simulink model "estimator_test_basic"  (R2018b)
settings: Solver=FixedStepAuto  StartTime=0.0  StopTime=1500  FixedStep=sim_params.sample_time_s  MaxStep=sim_params.sample_time_s  MinStep=sim_params.sample_time_s  RelTol=1e-5
undefined symbols (not defined in the file or in its folder): DiscIntNeverNeededParam, fsw_params, gyro_sim_lib, gyroscope_lib, magnetometer_lib, magnetometer_processing_lib, magnetometer_sim_lib, sensor_processing_libs, sim_params, sun_sensor_lib, sunsensor_processing_lib
libraries: vrlib x7, simulink x7, aerolibutil x5, dspmathops x2, simulink_extras x2, extended_kalman_filter_lib x1, ss_vec_2_angles x1, ss_angles_2_vec x1, dynamics_lib x1
settings Model: Creator=Taylor  LastModifiedBy=Taylor
settings SolverCC: InitialStep=sim_params.sample_time_s  InsertRTBMode=Always

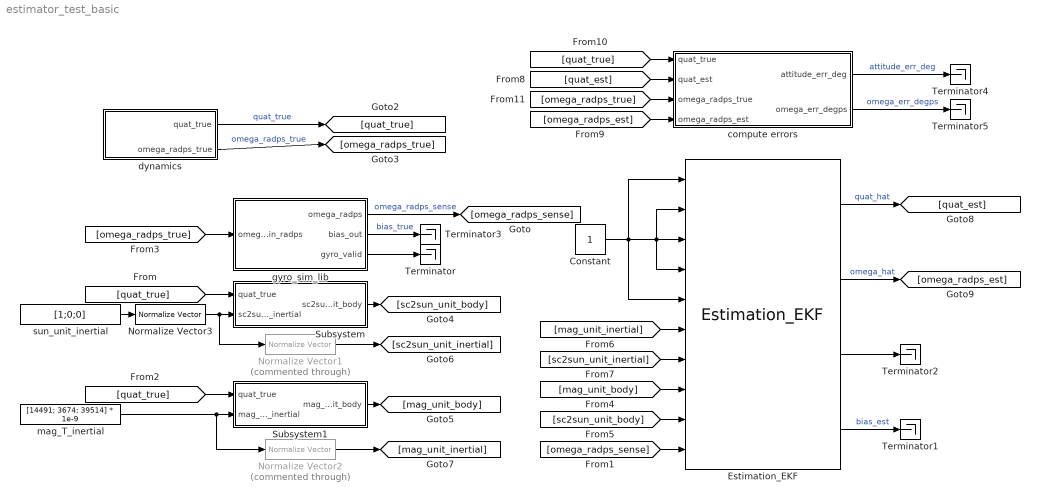
== system estimator_test_basic ==
  Constant : Constant
  "Estimation_EKF " : extended_kalman_filter_lib/Estimation_EKF   SystemSampleTime=-1
  Normalize Vector1 : vrlib/Utilities/Normalize Vector  Commented=through  maxzero=0
      settings: SourceProductName=Simulink 3D Animation  SourceProductBaseCode=VR
  Normalize Vector2 : vrlib/Utilities/Normalize Vector  Commented=through  maxzero=0
      settings: SourceProductName=Simulink 3D Animation  SourceProductBaseCode=VR
  Normalize Vector3 : vrlib/Utilities/Normalize Vector  maxzero=0
      settings: SourceProductName=Simulink 3D Animation  SourceProductBaseCode=VR
  Subsystem : Subsystem
  Subsystem1 : Subsystem
  Terminator{,1..5} (6 alike) : Terminator
  compute errors : Subsystem
  dynamics : Subsystem
  gyro_sim_lib : Subsystem  AncestorBlock=gyroscope_lib/gyro_sim_lib
  "mag_T_inertial " : Constant  Value=[14491; 3674; 39514] * 1e-9
  sun_unit_inertial : Constant  Value=[1;0;0]
  wires:
  Constant/1 -> "Estimation_EKF "/5, "Estimation_EKF "/1, "Estimation_EKF "/2, "Estimation_EKF "/4, "Estimation_EKF "/3
  gyro_sim_lib/1(omega_radps) -> [omega_radps_sense]  "omega_radps_sense"
  [omega_radps_sense] -> "Estimation_EKF "/10
  gyro_sim_lib/2(bias_out) -> Terminator3/1  "bias_true"
  gyro_sim_lib/3(gyro_valid) -> Terminator/1
  Subsystem/1(sc2sun_unit_body) -> [sc2sun_unit_body]
  Subsystem1/1(mag_unit_body) -> [mag_unit_body]
  dynamics/1(quat_true) -> [quat_true]  "quat_true"
  dynamics/2(omega_radps_true) -> [omega_radps_true]  "omega_radps_true"
  [quat_true] -> Subsystem/1(quat_true)
  [quat_true] -> Subsystem1/1(quat_true)
  [omega_radps_true] -> gyro_sim_lib/1(omega_in_radps)
  [mag_unit_body] -> "Estimation_EKF "/8
  [sc2sun_unit_body] -> "Estimation_EKF "/9
  "mag_T_inertial "/1 -> Normalize Vector2/1, Subsystem1/2(mag_T_inertial)
  [mag_unit_inertial] -> "Estimation_EKF "/6
  [sc2sun_unit_inertial] -> "Estimation_EKF "/7
  Normalize Vector1/1 -> [sc2sun_unit_inertial]
  "Estimation_EKF "/2 -> [omega_radps_est]  "omega_hat"
  "Estimation_EKF "/3 -> Terminator2/1
  "Estimation_EKF "/4 -> Terminator1/1  "bias_est"
  [quat_est] -> compute errors/2(quat_est)
  [omega_radps_est] -> compute errors/4(omega_radps_est)
  [quat_true] -> compute errors/1(quat_true)
  [omega_radps_true] -> compute errors/3(omega_radps_true)
  compute errors/1(attitude_err_deg) -> Terminator4/1  "attitude_err_deg"
  compute errors/2(omega_err_degps) -> Terminator5/1  "omega_err_degps"
  "Estimation_EKF "/1 -> [quat_est]  "quat_hat"
  Normalize Vector2/1 -> [mag_unit_inertial]
  Normalize Vector3/1 -> Normalize Vector1/1, Subsystem/2(sc2sun_unit_inertial)
  sun_unit_inertial/1 -> Normalize Vector3/1

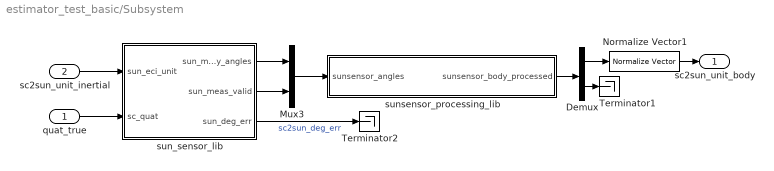
== system estimator_test_basic/Subsystem ==
  quat_true : Inport
  sc2sun_unit_inertial : Inport  Port=2
  Demux : Demux  Outputs=[3 1]
  Mux3 : Mux  Inputs=[2 1]
  Normalize Vector1 : vrlib/Utilities/Normalize Vector  maxzero=0
      settings: SourceProductName=Simulink 3D Animation  SourceProductBaseCode=VR
  Terminator1 : Terminator
  Terminator2 : Terminator
  sun_sensor_lib : Subsystem  AncestorBlock=sun_sensor_lib/sun_sensor_lib
  sunsensor_processing_lib : Subsystem  AncestorBlock=sensor_processing_libs/sunsensor_processing_lib
  sc2sun_unit_body : Outport
  wires:
  quat_true/1 -> sun_sensor_lib/2(sc_quat)
  sc2sun_unit_inertial/1 -> sun_sensor_lib/1(sun_eci_unit)
  sun_sensor_lib/3(sun_deg_err) -> Terminator2/1  "sc2sun_deg_err"
  sunsensor_processing_lib/1(sunsensor_body_processed) -> Demux/1
  sun_sensor_lib/1(sun_meas_body_angles) -> Mux3/1
  Mux3/1 -> sunsensor_processing_lib/1(sunsensor_angles)
  sun_sensor_lib/2(sun_meas_valid) -> Mux3/2
  Demux/1 -> Normalize Vector1/1
  Demux/2 -> Terminator1/1
  Normalize Vector1/1 -> sc2sun_unit_body/1

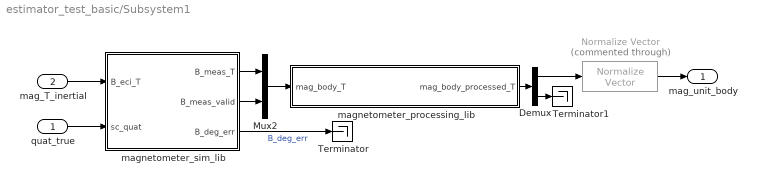
== system estimator_test_basic/Subsystem1 ==
  quat_true : Inport
  mag_T_inertial : Inport  Port=2
  Demux : Demux  Outputs=[3 1]
  Mux2 : Mux  Inputs=[3 1]
  Normalize Vector : vrlib/Utilities/Normalize Vector  Commented=through  maxzero=0
      settings: SourceProductName=Simulink 3D Animation  SourceProductBaseCode=VR
  Terminator : Terminator
  Terminator1 : Terminator
  magnetometer_processing_lib : Subsystem  AncestorBlock=sensor_processing_libs/magnetometer_processing_lib
  magnetometer_sim_lib : Subsystem  AncestorBlock=magnetometer_lib/magnetometer_sim_lib
  mag_unit_body : Outport
  wires:
  quat_true/1 -> magnetometer_sim_lib/2(sc_quat)
  mag_T_inertial/1 -> magnetometer_sim_lib/1(B_eci_T)
  magnetometer_sim_lib/2(B_meas_valid) -> Mux2/2
  magnetometer_sim_lib/1(B_meas_T) -> Mux2/1
  Mux2/1 -> magnetometer_processing_lib/1(mag_body_T)
  magnetometer_sim_lib/3(B_deg_err) -> Terminator/1  "B_deg_err"
  magnetometer_processing_lib/1(mag_body_processed_T) -> Demux/1
  Normalize Vector/1 -> mag_unit_body/1
  Demux/1 -> Normalize Vector/1
  Demux/2 -> Terminator1/1

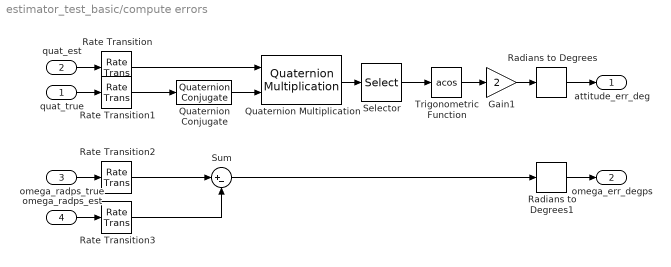
== system estimator_test_basic/compute errors ==
  quat_true : Inport
  quat_est : Inport  Port=2
  omega_radps_true : Inport  Port=3
  omega_radps_est : Inport  Port=4
  Gain1 : Gain  Gain=2
  Quaternion Conjugate : aerolibutil/Quaternion Conjugate
      settings: SourceProductName=Aerospace Blockset  SourceProductBaseCode=AE
  Quaternion Multiplication : aerolibutil/Quaternion Multiplication
  Radians to Degrees : simulink_extras/Transformations/Radians to Degrees
  Radians to Degrees1 : simulink_extras/Transformations/Radians to Degrees
  Rate Transition : RateTransition  InitialCondition=[1;0;0;0]  OutPortSampleTime=fsw_params.estimation.sample_time_s
  Rate Transition1 : RateTransition  InitialCondition=[1;0;0;0]  OutPortSampleTime=fsw_params.estimation.sample_time_s
  Rate Transition2 : RateTransition  OutPortSampleTime=fsw_params.estimation.sample_time_s
  Rate Transition3 : RateTransition  OutPortSampleTime=fsw_params.estimation.sample_time_s
  Selector : Selector  InputPortWidth=4  IndexOptions=Index vector (dialog)  Indices=[1]  OutputSizes=1
  Sum : Sum  Inputs=|+-
  Trigonometric Function : Trigonometry  Operator=acos
  attitude_err_deg : Outport
  omega_err_degps : Outport  Port=2
  wires:
  quat_true/1 -> Rate Transition1/1
  Selector/1 -> Trigonometric Function/1
  Trigonometric Function/1 -> Gain1/1
  Gain1/1 -> Radians to Degrees/1
  Quaternion Multiplication/1 -> Selector/1
  Radians to Degrees/1 -> attitude_err_deg/1
  omega_radps_true/1 -> Rate Transition2/1
  omega_radps_est/1 -> Rate Transition3/1
  Sum/1 -> Radians to Degrees1/1
  Radians to Degrees1/1 -> omega_err_degps/1
  Quaternion Conjugate/1 -> Quaternion Multiplication/2
  quat_est/1 -> Rate Transition/1
  Rate Transition/1 -> Quaternion Multiplication/1
  Rate Transition1/1 -> Quaternion Conjugate/1
  Rate Transition2/1 -> Sum/1
  Rate Transition3/1 -> Sum/2

== system estimator_test_basic/dynamics ==
  Constant : Constant  Commented=on  Value=zeros(3,1)
  Constant1 : Constant  Commented=on  Value=zeros(3,1)
  Constant2 : Constant  Value=[0.1;0;0]
  RigidBodyDynamics : Subsystem  Commented=on  AncestorBlock=dynamics_lib/Dynamics/RigidBodyDynamics
  quat_propagation : dynamics_lib/Dynamics/quat_propagation  SystemSampleTime=-1
  quat_true : Outport
  omega_radps_true : Outport  Port=2
  wires:
  quat_propagation/1 -> quat_true/1
  Constant/1 -> RigidBodyDynamics/1(external_torque)
  Constant1/1 -> RigidBodyDynamics/2(RW_torque)
  Constant2/1 -> omega_radps_true/1, quat_propagation/1

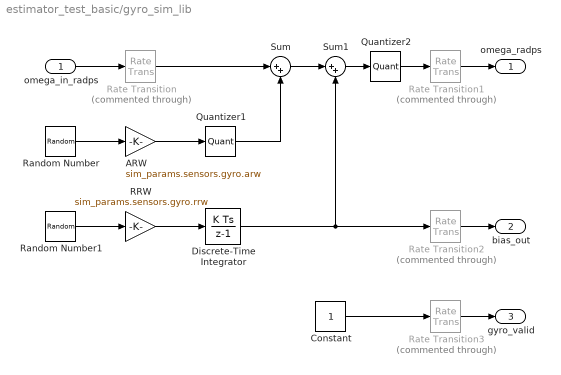
== system estimator_test_basic/gyro_sim_lib ==
  omega_in_radps : Inport
  ARW : Gain  Gain=sim_params.sensors.gyro.arw
  Constant : Constant  SampleTime=sim_params.sensors.gyro.sample_time_s
  Discrete-Time Integrator : DiscreteIntegrator  InitialCondition=sim_params.sensors.gyro.bias_init  SampleTime=-1  ICPrevOutput=DiscIntNeverNeededParam  ICPrevScaledInput=DiscIntNeverNeededParam
  Quantizer1 : Quantizer  QuantizationInterval=sim_params.sensors.gyro.resolution
  Quantizer2 : Quantizer  QuantizationInterval=sim_params.sensors.gyro.resolution
  RRW : Gain  Gain=sim_params.sensors.gyro.rrw
  Random Number : RandomNumber  Mean=[0 0 0]  Variance=[1 1 1]  Seed=[77 88 99]  SampleTime=sim_params.sensors.gyro.sample_time_s
  Random Number1 : RandomNumber  Mean=[0 0 0]  Variance=[1 1 1]  Seed=[81 82 83]  SampleTime=sim_params.sensors.gyro.sample_time_s
  Rate Transition : RateTransition  Commented=through  InitialCondition=sim_params.dynamics.ic.rate_init  OutPortSampleTime=sim_params.sensors.gyro.sample_time_s
  Rate Transition1 : RateTransition  Commented=through  InitialCondition=sim_params.dynamics.ic.rate_init
  Rate Transition2 : RateTransition  Commented=through  InitialCondition=sim_params.sensors.gyro.bias_init
  Rate Transition3 : RateTransition  Commented=through  InitialCondition=1
  Sum : Sum  Inputs=|++
  Sum1 : Sum  Inputs=|++
  omega_radps : Outport
  bias_out : Outport  Port=2
  gyro_valid : Outport  Port=3
  wires:
  Rate Transition3/1 -> gyro_valid/1
  Rate Transition2/1 -> bias_out/1
  Rate Transition1/1 -> omega_radps/1
  Rate Transition/1 -> Sum/1
  Quantizer2/1 -> Rate Transition1/1
  Sum1/1 -> Quantizer2/1
  Discrete-Time Integrator/1 -> Sum1/2, Rate Transition2/1
  Constant/1 -> Rate Transition3/1
  RRW/1 -> Discrete-Time Integrator/1
  Sum/1 -> Sum1/1
  omega_in_radps/1 -> Rate Transition/1
  ARW/1 -> Quantizer1/1
  Random Number1/1 -> RRW/1
  Random Number/1 -> ARW/1
  Quantizer1/1 -> Sum/2

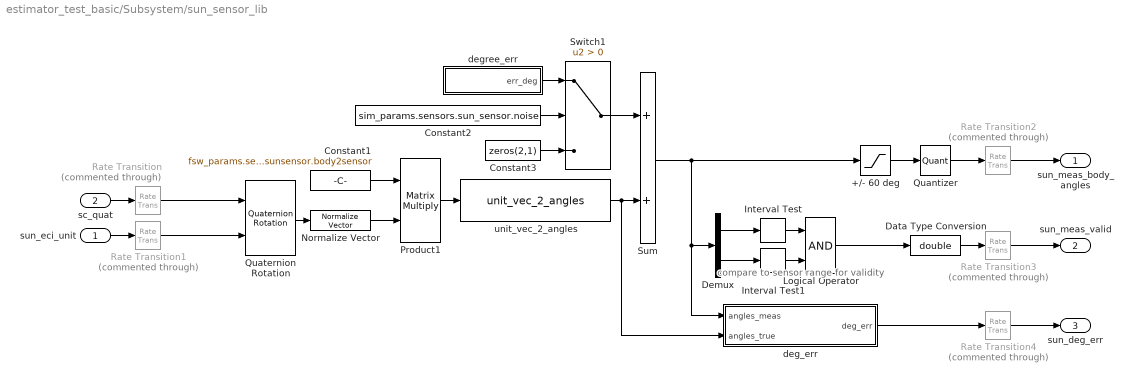
== system estimator_test_basic/Subsystem/sun_sensor_lib ==
  note: compare to sensor range for validity
  sun_eci_unit : Inport
  sc_quat : Inport  Port=2
  +/- 60 deg : Saturate  UpperLimit=60  LowerLimit=-60
  Constant1 : Constant  Value=fsw_params.sensor_processing.sunsensor.body2sensor  SampleTime=sim_params.sensors.sun_sensor.sample_time_s
  Constant2 : Constant  Value=sim_params.sensors.sun_sensor.noise  SampleTime=sim_params.sensors.sun_sensor.sample_time_s
  Constant3 : Constant  Value=zeros(2,1)  SampleTime=sim_params.sensors.sun_sensor.sample_time_s
  Data Type Conversion : DataTypeConversion  OutDataTypeStr=double
  Demux : Demux  Outputs=2
  Interval Test : simulink/Logic and Bit Operations/Interval Test  IntervalClosedRight=on  uplimit=sim_params.sensors.sun_sensor.range_deg  IntervalClosedLeft=on  lowlimit=-sim_params.sensors.sun_sensor.range_deg  OutDataTypeStr=boolean
  Interval Test1 : simulink/Logic and Bit Operations/Interval Test  IntervalClosedRight=on  uplimit=sim_params.sensors.sun_sensor.range_deg  IntervalClosedLeft=on  lowlimit=-sim_params.sensors.sun_sensor.range_deg  OutDataTypeStr=boolean
  Logical Operator : Logic  AllPortsSameDT=off  OutDataTypeStr=boolean
  Normalize Vector : vrlib/Utilities/Normalize Vector  maxzero=0
      settings: SourceProductName=Simulink 3D Animation  SourceProductBaseCode=VR
  Product1 : Product  Multiplication=Matrix(*)  RndMeth=Zero
  Quantizer : Quantizer  QuantizationInterval=sim_params.sensors.sun_sensor.resolution
  Quaternion Rotation : aerolibutil/Quaternion Rotation
  Rate Transition : RateTransition  Commented=through  InitialCondition=sim_params.dynamics.ic.quat_init  OutPortSampleTime=sim_params.sensors.sun_sensor.sample_time_s
  Rate Transition1 : RateTransition  Commented=through  OutPortSampleTime=sim_params.sensors.sun_sensor.sample_time_s
  Rate Transition2 : RateTransition  Commented=through
  Rate Transition3 : RateTransition  Commented=through
  Rate Transition4 : RateTransition  Commented=through
  Sum : Sum
  Switch1 : Switch  Criteria=u2 > Threshold
  deg_err : Subsystem
  degree_err : Subsystem
  unit_vec_2_angles : ss_vec_2_angles/unit_vec_2_angles  SystemSampleTime=-1
  sun_meas_body_angles : Outport
  sun_meas_valid : Outport  Port=2
  sun_deg_err : Outport  Port=3
  wires:
  Rate Transition4/1 -> sun_deg_err/1
  Rate Transition3/1 -> sun_meas_valid/1
  Rate Transition2/1 -> sun_meas_body_angles/1
  Rate Transition1/1 -> Quaternion Rotation/2
  Rate Transition/1 -> Quaternion Rotation/1
  Data Type Conversion/1 -> Rate Transition3/1
  Demux/2 -> Interval Test1/1
  Sum/1 -> Demux/1, deg_err/1(angles_meas), +/- 60 deg/1
  unit_vec_2_angles/1 -> Sum/2, deg_err/2(angles_true)
  Product1/1 -> unit_vec_2_angles/1
  Constant1/1 -> Product1/1
  +/- 60 deg/1 -> Quantizer/1
  Logical Operator/1 -> Data Type Conversion/1
  Interval Test1/1 -> Logical Operator/2
  Interval Test/1 -> Logical Operator/1
  Demux/1 -> Interval Test/1
  Normalize Vector/1 -> Product1/2
  Quantizer/1 -> Rate Transition2/1
  Quaternion Rotation/1 -> Normalize Vector/1
  degree_err/1("err_deg ") -> Switch1/1
  deg_err/1(deg_err) -> Rate Transition4/1
  sun_eci_unit/1 -> Rate Transition1/1
  Switch1/1 -> Sum/1
  Constant3/1 -> Switch1/3
  Constant2/1 -> Switch1/2
  sc_quat/1 -> Rate Transition/1

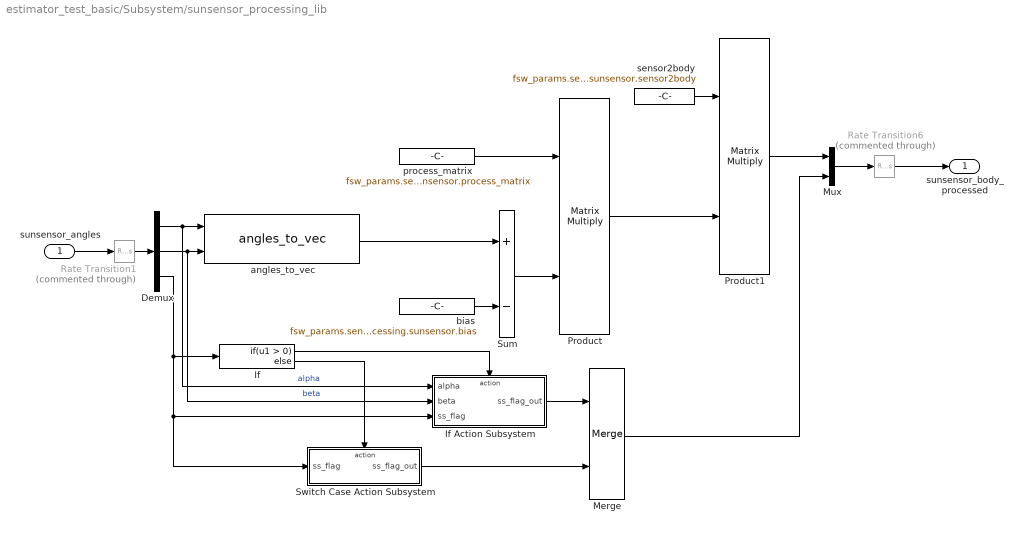
== system estimator_test_basic/Subsystem/sunsensor_processing_lib ==
  sunsensor_angles : Inport
  Demux : Demux  Outputs=[1 1 1]
  If : If
  If Action Subsystem : Subsystem  TreatAsAtomicUnit=on
  Merge : Merge
  Mux : Mux  Inputs=[3 1]
  Product : Product  Multiplication=Matrix(*)
  Product1 : Product  Multiplication=Matrix(*)
  Rate Transition1 : RateTransition  Commented=through  InitialCondition=fsw_params.sensor_processing.sunsensor.ic.angles  OutPortSampleTime=fsw_params.sensor_processing.sunsensor.sample_time_s
  Rate Transition6 : RateTransition  Commented=through
  Sum : Sum  Inputs=+-
  Switch Case Action Subsystem : Subsystem  TreatAsAtomicUnit=on
  angles_to_vec : ss_angles_2_vec/angles_to_vec  SystemSampleTime=-1
  bias : Constant  Value=fsw_params.sensor_processing.sunsensor.bias  SampleTime=fsw_params.sensor_processing.sunsensor.sample_time_s
  process_matrix : Constant  Value=fsw_params.sensor_processing.sunsensor.process_matrix  SampleTime=fsw_params.sensor_processing.sunsensor.sample_time_s
  sensor2body : Constant  Value=fsw_params.sensor_processing.sunsensor.sensor2body  SampleTime=fsw_params.sensor_processing.sunsensor.sample_time_s
  sunsensor_body_processed : Outport
  wires:
  process_matrix/1 -> Product/1
  Sum/1 -> Product/2
  Product/1 -> Product1/2
  bias/1 -> Sum/2
  sunsensor_angles/1 -> Rate Transition1/1
  sensor2body/1 -> Product1/1
  Product1/1 -> Mux/1
  Mux/1 -> Rate Transition6/1
  Rate Transition1/1 -> Demux/1
  Rate Transition6/1 -> sunsensor_body_processed/1
  Demux/1 -> If Action Subsystem/1(alpha), angles_to_vec/1  "alpha"
  Demux/2 -> If Action Subsystem/2(beta), angles_to_vec/2  "beta"
  angles_to_vec/1 -> Sum/1
  Merge/1 -> Mux/2
  Demux/3 -> If Action Subsystem/3(ss_flag), Switch Case Action Subsystem/1(ss_flag), If/1
  If/1 -> If Action Subsystem/Action
  If/2 -> Switch Case Action Subsystem/Action
  If Action Subsystem/1(ss_flag_out) -> Merge/1
  Switch Case Action Subsystem/1(ss_flag_out) -> Merge/2

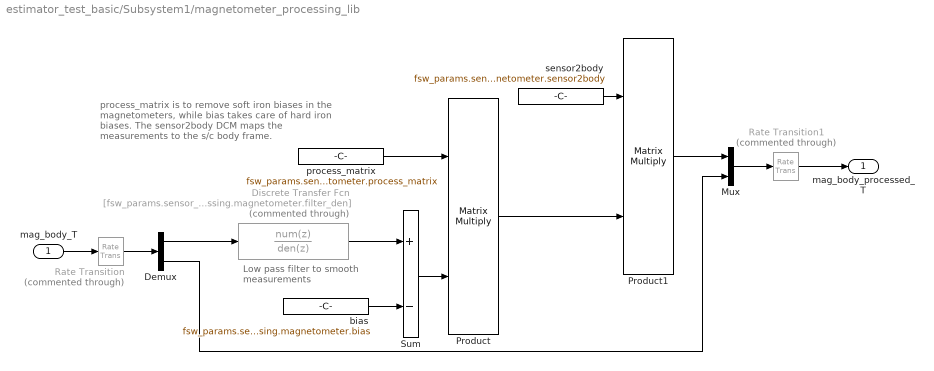
== system estimator_test_basic/Subsystem1/magnetometer_processing_lib ==
  note: Low pass filter to
      | smooth measurements
  note: process_matrix is to remove soft iron
      | biases in the magnetometers, while
      | bias takes care of hard iron biases.
      |
      | The sensor2body DCM maps the
      | measurements to the s/c body
      | frame.
  mag_body_T : Inport
  Demux : Demux  Outputs=[3 1]
  Discrete Transfer Fcn : DiscreteTransferFcn  Commented=through  Numerator=[fsw_params.sensor_processing.magnetometer.filter_num]  Denominator=[1 fsw_params.sensor_processing.magnetometer.filter_den]
  Mux : Mux  Inputs=[3 1]
  Product : Product  Multiplication=Matrix(*)
  Product1 : Product  Multiplication=Matrix(*)
  Rate Transition : RateTransition  Commented=through  OutPortSampleTime=fsw_params.sensor_processing.magnetometer.sample_time_s
  Rate Transition1 : RateTransition  Commented=through
  Sum : Sum  Inputs=+-
  bias : Constant  Value=fsw_params.sensor_processing.magnetometer.bias  SampleTime=fsw_params.sensor_processing.magnetometer.sample_time_s
  process_matrix : Constant  Value=fsw_params.sensor_processing.magnetometer.process_matrix  SampleTime=fsw_params.sensor_processing.magnetometer.sample_time_s
  sensor2body : Constant  Value=fsw_params.sensor_processing.magnetometer.sensor2body  SampleTime=fsw_params.sensor_processing.magnetometer.sample_time_s
  mag_body_processed_T : Outport
  wires:
  Discrete Transfer Fcn/1 -> Sum/1
  Rate Transition1/1 -> mag_body_processed_T/1
  Rate Transition/1 -> Demux/1
  Product1/1 -> Mux/1
  sensor2body/1 -> Product1/1
  Product/1 -> Product1/2
  Mux/1 -> Rate Transition1/1
  Demux/2 -> Mux/2
  Demux/1 -> Discrete Transfer Fcn/1
  process_matrix/1 -> Product/1
  Sum/1 -> Product/2
  bias/1 -> Sum/2
  mag_body_T/1 -> Rate Transition/1

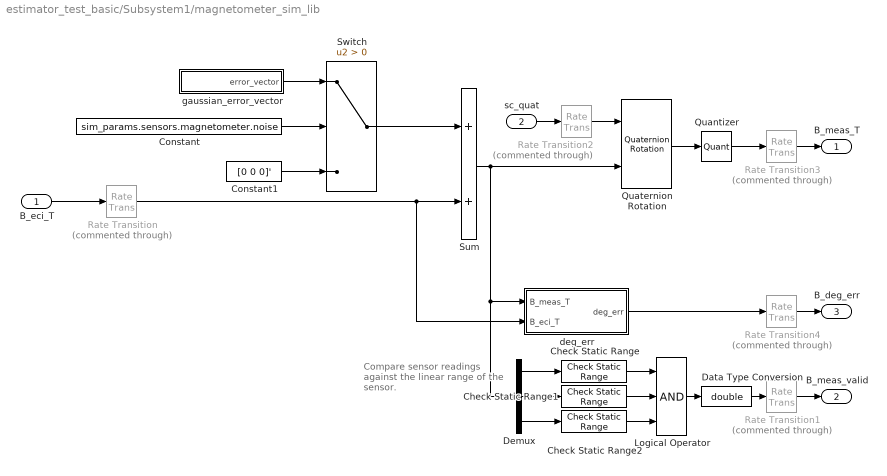
== system estimator_test_basic/Subsystem1/magnetometer_sim_lib ==
  note: Compare sensor readings
      | against the linear range
      | of the sensor.
  B_eci_T : Inport
  sc_quat : Inport  Port=2
  Check Static Range : simulink/Model Verification/Check  Static Range  Description=sim_params.sensors.magnetometer.B_min <= u <= sim_params.sensors.magnetometer.B_max  max=sim_params.sensors.magnetometer.B_max  max_included=on  min=sim_params.sensors.magnetometer.B_min  min_included=on  enabled=on  stopWhenAssertionFail=off  export=on  icon=text
      settings: SourceProductName=Simulink  SourceProductBaseCode=SL
  Check Static Range1 : simulink/Model Verification/Check  Static Range  Description=sim_params.sensors.magnetometer.B_min <= u <= sim_params.sensors.magnetometer.B_max  max=sim_params.sensors.magnetometer.B_max  max_included=on  min=sim_params.sensors.magnetometer.B_min  min_included=on  enabled=on  stopWhenAssertionFail=off  export=on  icon=graphic
      settings: SourceProductName=Simulink  SourceProductBaseCode=SL
  Check Static Range2 : simulink/Model Verification/Check  Static Range  Description=sim_params.sensors.magnetometer.B_min <= u <= sim_params.sensors.magnetometer.B_max  max=sim_params.sensors.magnetometer.B_max  max_included=on  min=sim_params.sensors.magnetometer.B_min  min_included=on  enabled=on  stopWhenAssertionFail=off  export=on  icon=graphic
      settings: SourceProductName=Simulink  SourceProductBaseCode=SL
  Constant : Constant  Value=sim_params.sensors.magnetometer.noise  SampleTime=sim_params.sensors.magnetometer.sample_time_s
  Constant1 : Constant  Value=[0 0 0]'  SampleTime=sim_params.sensors.magnetometer.sample_time_s
  Data Type Conversion : DataTypeConversion  OutDataTypeStr=double
  Demux : Demux  Outputs=3
  Logical Operator : Logic  Inputs=3  AllPortsSameDT=off  OutDataTypeStr=boolean
  Quantizer : Quantizer  QuantizationInterval=sim_params.sensors.magnetometer.resolution
  Quaternion Rotation : aerolibutil/Quaternion Rotation
  Rate Transition : RateTransition  Commented=through  InitialCondition=sim_params.environment.magnetic.ic.eci_T  OutPortSampleTime=sim_params.sensors.magnetometer.sample_time_s
  Rate Transition1 : RateTransition  Commented=through
  Rate Transition2 : RateTransition  Commented=through  InitialCondition=sim_params.dynamics.ic.quat_init  OutPortSampleTime=sim_params.sensors.magnetometer.sample_time_s
  Rate Transition3 : RateTransition  Commented=through  InitialCondition=sim_params.environment.magnetic.ic.eci_T
  Rate Transition4 : RateTransition  Commented=through
  Sum : Sum
  Switch : Switch  Criteria=u2 > Threshold
  deg_err : Subsystem
  gaussian_error_vector : Subsystem
  B_meas_T : Outport
  B_meas_valid : Outport  Port=2
  B_deg_err : Outport  Port=3
  wires:
  Data Type Conversion/1 -> Rate Transition1/1
  Logical Operator/1 -> Data Type Conversion/1
  Check Static Range2/1 -> Logical Operator/3
  Check Static Range1/1 -> Logical Operator/2
  Check Static Range/1 -> Logical Operator/1
  Demux/3 -> Check Static Range2/1
  Demux/2 -> Check Static Range1/1
  Demux/1 -> Check Static Range/1
  Quantizer/1 -> Rate Transition3/1
  Rate Transition4/1 -> B_deg_err/1
  Quaternion Rotation/1 -> Quantizer/1
  Rate Transition3/1 -> B_meas_T/1
  Rate Transition2/1 -> Quaternion Rotation/1
  Rate Transition1/1 -> B_meas_valid/1
  Rate Transition/1 -> Sum/2, deg_err/2(B_eci_T)
  deg_err/1(deg_err) -> Rate Transition4/1
  B_eci_T/1 -> Rate Transition/1
  gaussian_error_vector/1(error_vector) -> Switch/1
  Constant1/1 -> Switch/3
  Sum/1 -> Demux/1, deg_err/1(B_meas_T), Quaternion Rotation/2
  Constant/1 -> Switch/2
  Switch/1 -> Sum/1
  sc_quat/1 -> Rate Transition2/1

== system estimator_test_basic/dynamics/RigidBodyDynamics ==
  external_torque : Inport
  RW_torque : Inport  Port=2
  Discrete-Time Integrator : DiscreteIntegrator  InitialCondition=[0;0;0]  SampleTime=-1  ICPrevOutput=DiscIntNeverNeededParam  ICPrevScaledInput=DiscIntNeverNeededParam
  "Discrete-Time Integrator " : DiscreteIntegrator  InitialCondition=[0.1;0.05;-0.07]  SampleTime=-1  ICPrevOutput=DiscIntNeverNeededParam  ICPrevScaledInput=DiscIntNeverNeededParam
  dynamics : Subsystem
  body_rates : Outport
  wires:
  RW_torque/1 -> dynamics/2(rw_torque_Nm), Discrete-Time Integrator/1
  Discrete-Time Integrator/1 -> dynamics/3(rw_momentum_Nms)
  "Discrete-Time Integrator "/1 -> body_rates/1, dynamics/4(omega_radps)
  external_torque/1 -> dynamics/1(external_torque_Nm)
  dynamics/1(omega_dot) -> "Discrete-Time Integrator "/1

== system estimator_test_basic/Subsystem/sun_sensor_lib/deg_err ==
  note: Computes the norm of the 2x1 degree error vector
  angles_meas : Inport
  angles_true : Inport  Port=2
  Dot Product : DotProduct  InputSameDT=on  OutDataTypeStr=Inherit: Inherit via internal rule
  Sqrt : Sqrt  SaturateOnIntegerOverflow=on
  Sum : Sum  Inputs=+-
  deg_err : Outport
  wires:
  Sqrt/1 -> deg_err/1
  Dot Product/1 -> Sqrt/1
  Sum/1 -> Dot Product/1, Dot Product/2
  angles_true/1 -> Sum/2
  angles_meas/1 -> Sum/1

== system estimator_test_basic/Subsystem/sun_sensor_lib/degree_err ==
  Mux : Mux  Inputs=2
  Random Number2 : RandomNumber  Variance=sim_params.sensors.sun_sensor.deg_err  Seed=51  SampleTime=sim_params.sensors.sun_sensor.sample_time_s
  Random Number3 : RandomNumber  Variance=sim_params.sensors.sun_sensor.deg_err  Seed=52  SampleTime=sim_params.sensors.sun_sensor.sample_time_s
  "err_deg " : Outport
  wires:
  Mux/1 -> "err_deg "/1
  Random Number3/1 -> Mux/2
  Random Number2/1 -> Mux/1

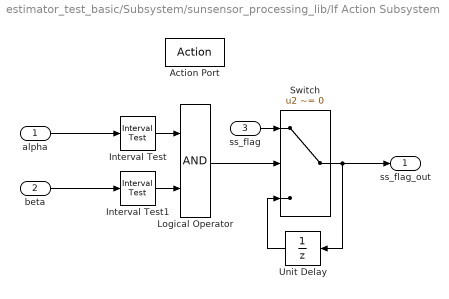
== system estimator_test_basic/Subsystem/sunsensor_processing_lib/If Action Subsystem ==
  alpha : Inport
  beta : Inport  Port=2
  ss_flag : Inport  Port=3
  Action Port : ActionPort  InitializeStates=reset  ActionType=then
  Interval Test : simulink/Logic and Bit Operations/Interval Test  IntervalClosedRight=on  uplimit=fsw_params.sensor_processing.sunsensor.ang_thresh  IntervalClosedLeft=on  lowlimit=-fsw_params.sensor_processing.sunsensor.ang_thresh  OutDataTypeStr=boolean
  Interval Test1 : simulink/Logic and Bit Operations/Interval Test  IntervalClosedRight=on  uplimit=fsw_params.sensor_processing.sunsensor.ang_thresh  IntervalClosedLeft=on  lowlimit=-fsw_params.sensor_processing.sunsensor.ang_thresh  OutDataTypeStr=boolean
  Logical Operator : Logic  AllPortsSameDT=off  OutDataTypeStr=boolean
  Switch : Switch  Criteria=u2 ~= 0
  Unit Delay : UnitDelay  InitialCondition=2  SampleTime=-1
  ss_flag_out : Outport
  wires:
  Switch/1 -> ss_flag_out/1, Unit Delay/1
  Interval Test/1 -> Logical Operator/1
  Interval Test1/1 -> Logical Operator/2
  beta/1 -> Interval Test1/1
  alpha/1 -> Interval Test/1
  ss_flag/1 -> Switch/1
  Logical Operator/1 -> Switch/2
  Unit Delay/1 -> Switch/3

== system estimator_test_basic/Subsystem/sunsensor_processing_lib/Switch Case Action Subsystem ==
  ss_flag : Inport
  Action Port : ActionPort  ActionType=else
  ss_flag_out : Outport
  wires:
  ss_flag/1 -> ss_flag_out/1

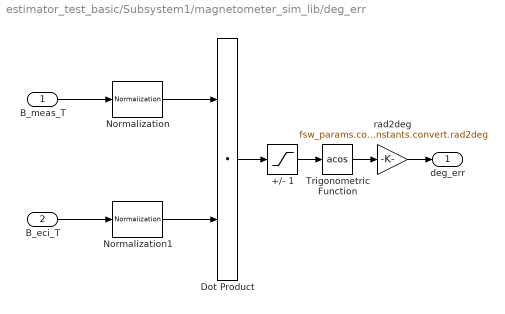
== system estimator_test_basic/Subsystem1/magnetometer_sim_lib/deg_err ==
  B_meas_T : Inport
  B_eci_T : Inport  Port=2
  +/- 1 : Saturate  UpperLimit=1  LowerLimit=-1
  Dot Product : DotProduct  InputSameDT=on  OutDataTypeStr=Inherit: Inherit via internal rule
  Normalization : dspmathops/Normalization  NormType=2-norm  Bias=1e-10  NormOver=Each column  Dimension=1  roundingMode=Floor  overflowMode=off  accumDataTypeStr=Inherit: Same as product output  accumLastDataTypeStr=Inherit: Same as product output  outputDataTypeStr=Inherit: Same as product output  outputMin=[]  outputMax=[]  outputLastDataTypeStr=Inherit: Same as product output
      settings: SourceProductName=DSP System Toolbox
  Normalization1 : dspmathops/Normalization  NormType=2-norm  Bias=1e-10  NormOver=Each column  Dimension=1  roundingMode=Floor  overflowMode=off  accumDataTypeStr=Inherit: Same as product output  accumLastDataTypeStr=Inherit: Same as product output  outputDataTypeStr=Inherit: Same as product output  outputMin=[]  outputMax=[]  outputLastDataTypeStr=Inherit: Same as product output
      settings: SourceProductName=DSP System Toolbox
  Trigonometric Function : Trigonometry  Operator=acos
  rad2deg : Gain  Gain=fsw_params.constants.convert.rad2deg
  deg_err : Outport
  wires:
  rad2deg/1 -> deg_err/1
  +/- 1/1 -> Trigonometric Function/1
  Trigonometric Function/1 -> rad2deg/1
  Dot Product/1 -> +/- 1/1
  Normalization1/1 -> Dot Product/2
  B_eci_T/1 -> Normalization1/1
  Normalization/1 -> Dot Product/1
  B_meas_T/1 -> Normalization/1

== system estimator_test_basic/Subsystem1/magnetometer_sim_lib/gaussian_error_vector ==
  Mux : Mux  Inputs=3
  Random Number2 : RandomNumber  Seed=4  SampleTime=sim_params.sensors.magnetometer.sample_time_s
  Random Number3 : RandomNumber  Seed=5  SampleTime=sim_params.sensors.magnetometer.sample_time_s
  Random Number4 : RandomNumber  Seed=6  SampleTime=sim_params.sensors.magnetometer.sample_time_s
  sigma_mag_x : Gain  Gain=sim_params.sensors.magnetometer.err_x
  sigma_mag_y : Gain  Gain=sim_params.sensors.magnetometer.err_y
  sigma_mag_z : Gain  Gain=sim_params.sensors.magnetometer.err_z
  error_vector : Outport
  wires:
  sigma_mag_z/1 -> Mux/3
  Mux/1 -> error_vector/1
  sigma_mag_y/1 -> Mux/2
  sigma_mag_x/1 -> Mux/1
  Random Number3/1 -> sigma_mag_y/1
  Random Number4/1 -> sigma_mag_z/1
  Random Number2/1 -> sigma_mag_x/1

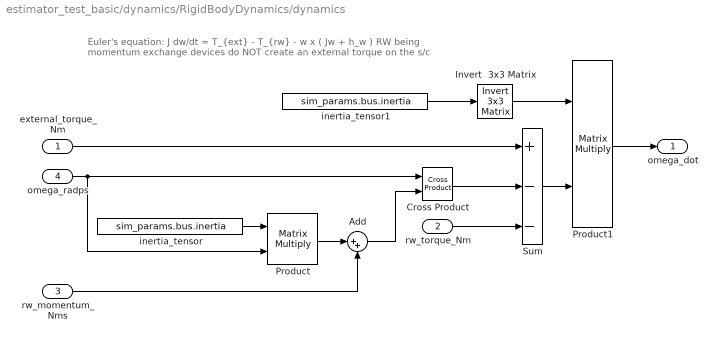
== system estimator_test_basic/dynamics/RigidBodyDynamics/dynamics ==
  note: Euler's equation: J dw/dt = T_{ext} - T_{rw} - w x ( Jw + h_w )
      |
      | RW being momentum exchange devices do NOT create
      | an external torque on the s/c
  external_torque_Nm : Inport
  rw_torque_Nm : Inport  Port=2
  rw_momentum_Nms : Inport  Port=3
  omega_radps : Inport  Port=4
  Add : Sum  Inputs=|++
  Cross Product : vrlib/Utilities/Cross Product
      settings: SourceProductBaseCode=VR
  Invert  3x3 Matrix : aerolibutil/Invert  3x3 Matrix
  Product : Product  Multiplication=Matrix(*)  RndMeth=Zero
  Product1 : Product  Multiplication=Matrix(*)  RndMeth=Zero
  Sum : Sum  Inputs=+--
  inertia_tensor : Constant  Value=sim_params.bus.inertia  SampleTime=sim_params.sample_time_s
  inertia_tensor1 : Constant  Value=sim_params.bus.inertia  SampleTime=sim_params.sample_time_s
  omega_dot : Outport
  wires:
  rw_torque_Nm/1 -> Sum/3
  Add/1 -> Cross Product/2
  rw_momentum_Nms/1 -> Add/2
  Product/1 -> Add/1
  Cross Product/1 -> Sum/2
  inertia_tensor1/1 -> Invert  3x3 Matrix/1
  Invert  3x3 Matrix/1 -> Product1/1
  Product1/1 -> omega_dot/1
  Sum/1 -> Product1/2
  inertia_tensor/1 -> Product/1
  omega_radps/1 -> Cross Product/1, Product/2
  external_torque_Nm/1 -> Sum/1
